simulink model "TrafficLIghtSyatem"  (R2020a)
settings: Solver=FixedStepDiscrete  StartTime=0.0  StopTime=150  FixedStep=0.1  RelTol=1e-3  EnableMultiTasking=on
model workspace (MAT data in the model file):
  GREEN = 1
undefined symbols (not defined in the file or in its folder): DiscIntNeverNeededParam
libraries: simulink x1
settings Model: Creator=Admin  LastModifiedBy=Admin

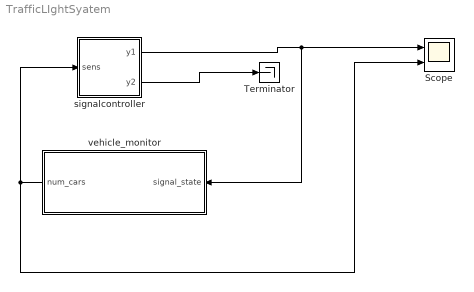
== system TrafficLIghtSyatem ==
  Scope : Scope  NumInputPorts=2
  Terminator : Terminator
  signalcontroller : Stateflow chart  TreatAsAtomicUnit=on
  vehicle_monitor : Subsystem
  wires:
  vehicle_monitor/1(num_cars) -> signalcontroller/1(sens), Scope/2
  signalcontroller/2(y2) -> Terminator/1
  signalcontroller/1(y1) -> vehicle_monitor/1(signal_state), Scope/1

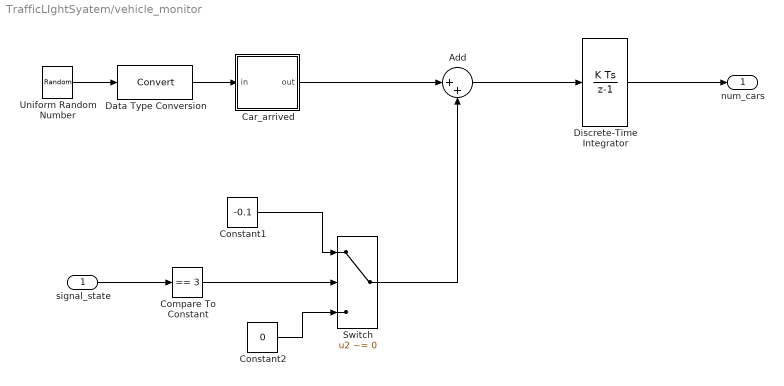
== system TrafficLIghtSyatem/vehicle_monitor ==
  signal_state : Inport
  Add : Sum  Inputs=|++
  Car_arrived : Stateflow chart  TreatAsAtomicUnit=on
  Compare To Constant : simulink/Logic and Bit Operations/Compare To Constant  relop===  const=3  OutDataTypeStr=boolean  ZeroCross=off
  Constant1 : Constant  Value=-0.1
  Constant2 : Constant  Value=0
  Data Type Conversion : DataTypeConversion
  Discrete-Time Integrator : DiscreteIntegrator  SampleTime=-1  LimitOutput=on  LowerSaturationLimit=0  ICPrevOutput=DiscIntNeverNeededParam  ICPrevScaledInput=DiscIntNeverNeededParam
  Switch : Switch  Criteria=u2 ~= 0
  Uniform Random Number : UniformRandomNumber  Minimum=0  Maximum=100  Seed=177836  SampleTime=0
  num_cars : Outport  VectorParamsAs1DForOutWhenUnconnected=off
  wires:
  Car_arrived/1(out) -> Add/1
  Switch/1 -> Add/2
  signal_state/1 -> Compare To Constant/1
  Discrete-Time Integrator/1 -> num_cars/1
  Uniform Random Number/1 -> Data Type Conversion/1
  Compare To Constant/1 -> Switch/2
  Data Type Conversion/1 -> Car_arrived/1(in)
  Constant1/1 -> Switch/1
  Add/1 -> Discrete-Time Integrator/1
  Constant2/1 -> Switch/3

== stateflow chart TrafficLIghtSyatem/signalcontroller ==
  state Stop
    y1 = RED;
    y2 = GREEN;
  state StopForTraffic
    y1 = RED;
    y2 = GREEN;
  state StopToGo
    y1 = RED;
    y2 = YELLOW;
  state GoToStop
    y1 = YELLOW;
    y2 = RED;
  state Go
    y1 = GREEN;
    y2 = RED;
  (default) -> Stop
  StopForTraffic -> StopToGo : [sens]
  Stop -> StopForTraffic : after(20,tick)
  GoToStop -> Stop : after (3,tick)
  StopToGo -> Go : after(3,tick)
  Go -> GoToStop : after(10,tick)
  data: sens input; y1 output double; y2 output double; GREEN constant double =3; RED constant double =1; YELLOW constant double =2

== stateflow chart TrafficLIghtSyatem/vehicle_monitor/Car_arrived ==
  (default) -> (junction 2) : {out = in > 98;}
  data: in input int8; out output double
